simulink model "driver_interface"  (R2022b)
settings: Solver=FixedStepAuto  StartTime=0.0  StopTime=10.0  FixedStep=1e-3  RelTol=1e-3
libraries: driver_interface_lib x1
settings Model: Creator=dr_pa  LastModifiedBy=dr_pa
settings DataIOCC: ExternalInput=DI2.getElement('GOV_e_diCmd'),DI2.getElement('DI_V_BrakePedalPos'),DI2.getElement('DI_b_DriverButton'),DI2.getElement('DI_V_AccelPedalPos1'),DI2.getElement('DI_V_AccelPedalPos2'),DI2.getElement('Dl_V_RawSteeringAngle')  LoadExternalInput=on

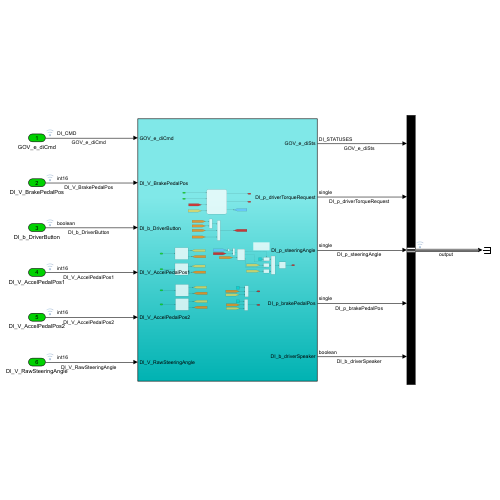
[thumbnail: Simulink's stored preview of the top-level diagram]
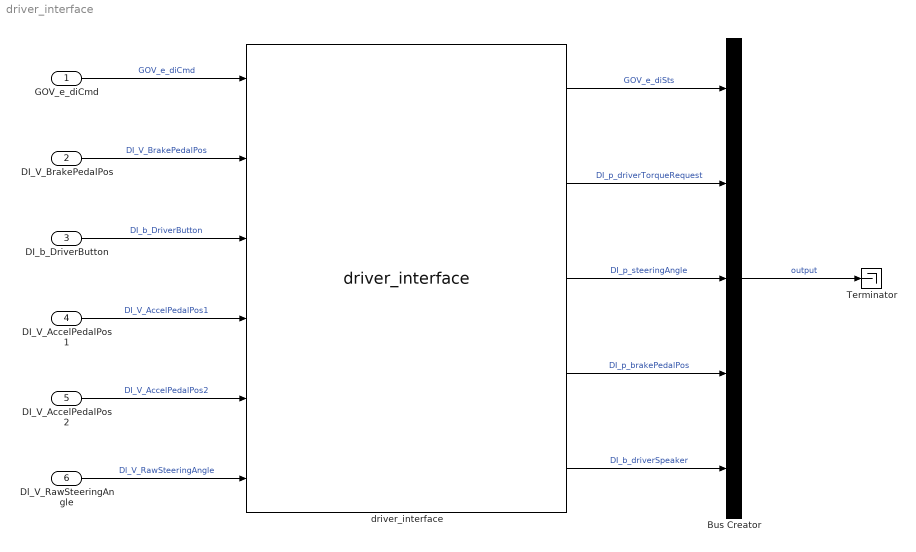
== system driver_interface ==
  GOV_e_diCmd : Inport  Interpolate=off
  DI_V_BrakePedalPos : Inport  Port=2
  DI_b_DriverButton : Inport  Port=3  OutDataTypeStr=boolean
  DI_V_AccelPedalPos1 : Inport  Port=4
  DI_V_AccelPedalPos2 : Inport  Port=5
  Dl_V_RawSteeringAngle : Inport  Port=6
  Bus Creator : BusCreator  Inputs=5
  Terminator : Terminator
  driver_interface : driver_interface_lib/driver_interface  SystemSampleTime=-1  VariantActivationTime=update diagram  Latency=0  AutoFrameSizeCalculation=off
  wires:
  Dl_V_RawSteeringAngle/1 -> driver_interface/6  "Dl_V_RawSteeringAngle"
  DI_V_BrakePedalPos/1 -> driver_interface/2  "DI_V_BrakePedalPos"
  GOV_e_diCmd/1 -> driver_interface/1  "GOV_e_diCmd"
  DI_V_AccelPedalPos1/1 -> driver_interface/4  "DI_V_AccelPedalPos1"
  DI_b_DriverButton/1 -> driver_interface/3  "DI_b_DriverButton"
  DI_V_AccelPedalPos2/1 -> driver_interface/5  "DI_V_AccelPedalPos2"
  driver_interface/2 -> Bus Creator/2  "DI_p_driverTorqueRequest"
  driver_interface/1 -> Bus Creator/1  "GOV_e_diSts"
  driver_interface/3 -> Bus Creator/3  "DI_p_steeringAngle"
  driver_interface/4 -> Bus Creator/4  "DI_p_brakePedalPos"
  driver_interface/5 -> Bus Creator/5  "DI_b_driverSpeaker"
  Bus Creator/1 -> Terminator/1  "output"
